simulink subsystem "heart_cycle"  (R2020b)
settings: Solver=VariableStepAuto  StartTime=0.0  StopTime=10.0  RelTol=1e-3
settings Model: Creator=RH  LastModifiedBy=Marco

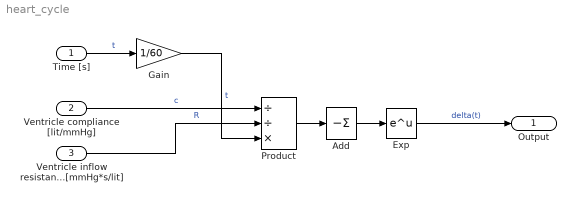
== system heart_cycle ==
  Time [s] : Inport  Unit=s
  Ventricle compliance [lit/mmHg] : Inport  Port=2  Unit=liter/mmHg
  Ventricle inflow resistance [mmHg*s/lit] : Inport  Port=3  Unit=mmHg*minute/liter
  Add : Sum  Inputs=-
  Exp : Math  SaturateOnIntegerOverflow=on
  Gain : Gain  Gain=1/60
  Product : Product  Inputs=//*
  Output : Outport  Unit=1
  wires:
  Ventricle compliance [lit/mmHg]/1 -> Product/1  "c"
  Ventricle inflow resistance [mmHg*s/lit]/1 -> Product/2  "R"
  Product/1 -> Add/1
  Add/1 -> Exp/1
  Exp/1 -> Output/1  "delta(t)"
  Time [s]/1 -> Gain/1  "t"
  Gain/1 -> Product/3  "t"
